simulink model "stepper_foc"  (R2021b)
settings: Solver=ode5  StartTime=0.0  StopTime=1  FixedStep=0.000001  MinStep=0.0001  RelTol=1e-3
InitFcn:
  | L=1.75e-3;
  | R=0.38;
  | Km=0.015;
  | Nr=50;
  | B=1e-3;
  | J=4.8e-5;
  | 
  | %%i_u_convert
  | K4=0.1;
  | 
  | b1=0.7;
  | b2=0.3;
  | b3=0.05;
  | b4=0;
undefined symbols (not defined in the file or in its folder): ia, ib, magnitude, Omega, Theta
settings Model: Creator=ACER  LastModifiedBy=ACER
settings SolverCC: MaxConsecutiveMinStep=10  AllowMultiTaskInputOutput=on  AutoInsertRateTranBlk=on
settings OptimizationCC: DefaultParameterBehavior=Inlined  UseDivisionForNetSlopeComputation=on  GainParamInheritBuiltInType=on  UseFloatMulNetSlope=on  InlineInvariantSignals=on  PassReuseOutputArgsAs=Individual arguments  ZeroExternalMemoryAtStartup=off  ZeroInternalMemoryAtStartup=off  NoFixptDivByZeroProtection=on  EfficientFloat2IntCast=on  LifeSpan=1  OptimizeBlockOrder=speed  DifferentSizesBufferReuse=on  EfficientTunableParamExpr=on
settings DebuggingCC: ParameterTunabilityLossMsg=error
settings HardwareCC: ProdBitPerInt=16  ProdBitPerPointer=16  ProdBitPerSizeT=16  ProdBitPerPtrDiffT=16  ProdLargestAtomicFloat=None  ProdWordSize=16  ProdLongLongMode=on  ProdHWDeviceType=STMicroelectronics->ST10/Super10
settings SFSimCC: MATLABDynamicMemAlloc=off
settings RTWCC: Description=Embedded Coder  SystemTargetFile=ert.tlc  TemplateMakefile=ert_default_tmf
settings CodeAppCC: ForceParamTrailComments=on  IgnoreCustomStorageClasses=off  OperatorAnnotations=on  SimulinkDataObjDesc=on  SFDataObjDesc=on  CustomSymbolStrGlobalVar=rt$N$M  CustomSymbolStrType=$N$M  CustomSymbolStrFcn=$N$M$F  CustomSymbolStrMacro=$N$M  InsertBlockDesc=on
settings ERTTargetCC: TargetLangStandard=C99 (ISO)  GenerateSampleERTMain=on  IncludeMdlTerminateFcn=off  CombineSignalStateStructs=on  SupportComplex=off  SupportContinuousTime=on  SupportNonInlinedSFcns=on  InlinedParameterPlacement=NonHierarchical  ERTCustomFileTemplate=example_file_process.tlc  ERTFilePackagingFormat=CompactWithDataFile

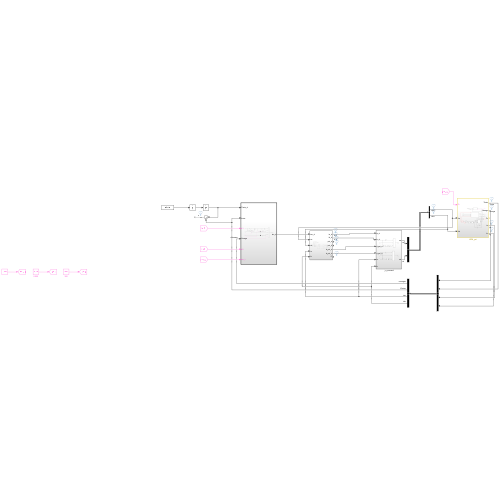
[thumbnail: Simulink's stored preview of the top-level diagram]
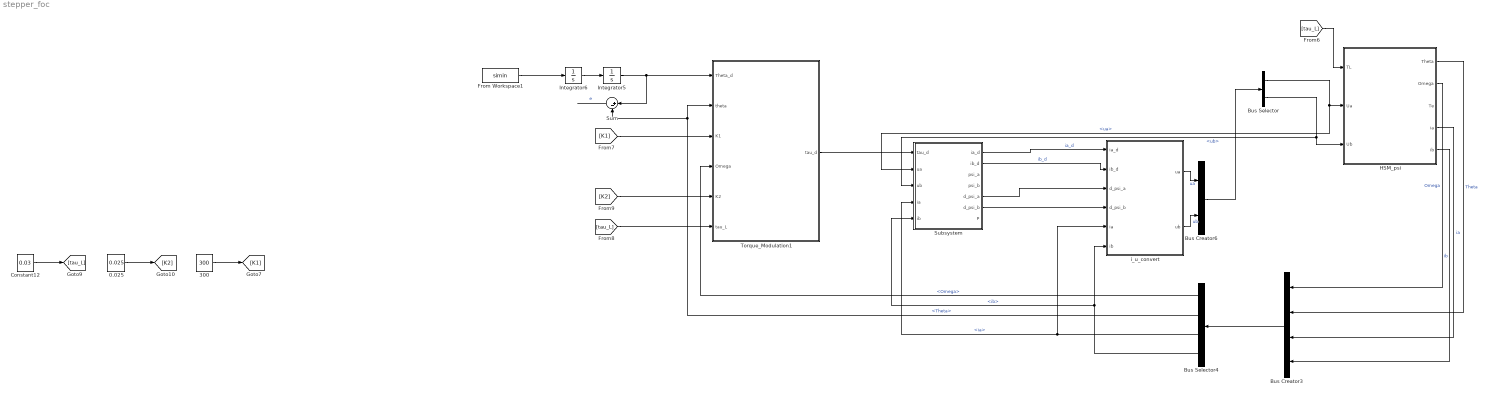
== system stepper_foc ==
  0.025 : Constant  Value=0.025
  300 : Constant  Value=300
  Bus Creator3 : BusCreator  Inputs=Omega,Theta,ia,ib
  Bus Creator6 : BusCreator  Inputs=2
  Bus Selector : BusSelector  OutputSignals=ua,ub
  Bus Selector4 : BusSelector  OutputSignals=Omega,Theta,ia,ib
  Constant12 : Constant  Value=0.03
  From Workspace1 : FromWorkspace  VariableName=simin  OutputAfterFinalValue=Holding final value
  HSM_psi : Subsystem  TreatAsAtomicUnit=on
      settings: MinAlgLoopOccurrences=on
  Integrator5 : Integrator
  Integrator6 : Integrator
  Subsystem : Subsystem
      settings: MinAlgLoopOccurrences=on
  Sum : Sum  Inputs=|+-
  Torque_Modulation1 : Subsystem  TreatAsAtomicUnit=on
  i_u_convert : Subsystem
      settings: MinAlgLoopOccurrences=on
  wires:
  Bus Creator3/1 -> Bus Selector4/1
  Integrator6/1 -> Integrator5/1
  [K2] -> Torque_Modulation1/5(K2)
  [K1] -> Torque_Modulation1/3(K1)
  Bus Selector4/1 -> Torque_Modulation1/4(Omega)  "<Omega>"
  Bus Selector4/2 -> Sum/2, Torque_Modulation1/2(theta)  "<Theta>"
  Bus Selector4/3 -> Subsystem/4(ia), i_u_convert/5(ia)  "<ia>"
  Bus Selector4/4 -> Subsystem/5(ib), i_u_convert/6(ib)  "<ib>"
  HSM_psi/4(ia) -> Bus Creator3/3  "ia"
  HSM_psi/5(ib) -> Bus Creator3/4  "ib"
  HSM_psi/1(Theta) -> Bus Creator3/2  "Theta"
  HSM_psi/2(Omega) -> Bus Creator3/1  "Omega"
  [tau_L] -> HSM_psi/1(TL)
  Bus Selector/1 -> Subsystem/2(ua), HSM_psi/2(Ua)  "<ua>"
  Bus Selector/2 -> HSM_psi/3(Ub), Subsystem/3(ub)  "<ub>"
  i_u_convert/1(ua) -> Bus Creator6/1  "ua"
  i_u_convert/2(ub) -> Bus Creator6/2  "ub"
  Subsystem/1(ia_d) -> i_u_convert/1(ia_d)  "ia_d"
  Integrator5/1 -> Sum/1, Torque_Modulation1/1(Theta_d)
  300/1 -> [K1]
  0.025/1 -> [K2]
  Constant12/1 -> [tau_L]
  Subsystem/2(ib_d) -> i_u_convert/2(ib_d)  "ib_d"
  Bus Creator6/1 -> Bus Selector/1
  Subsystem/5(d_psi_a) -> i_u_convert/3(d_psi_a)
  Subsystem/6(d_psi_b) -> i_u_convert/4(d_psi_b)
  [tau_L] -> Torque_Modulation1/6(tau_L)
  From Workspace1/1 -> Integrator6/1
  Torque_Modulation1/1(tau_d) -> Subsystem/1(tau_d)
  Sum/1 -> ?  "e"

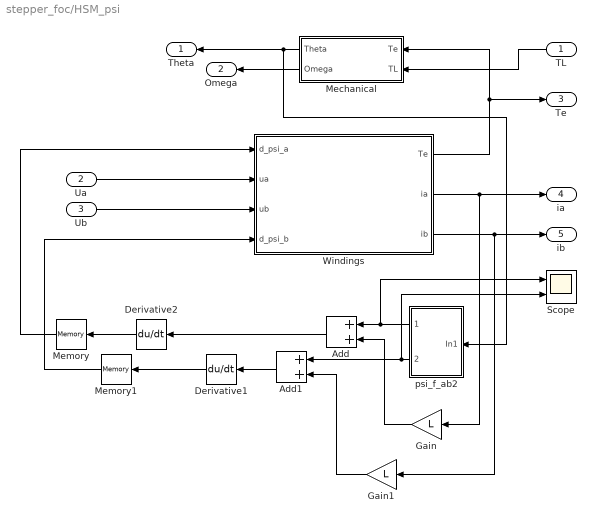
== system stepper_foc/HSM_psi ==
  TL : Inport
  Ua : Inport  Port=2
  Ub : Inport  Port=3
  Add : Sum
  Add1 : Sum
  Derivative1 : Derivative
  Derivative2 : Derivative
  Gain : Gain  Gain=L
  Gain1 : Gain  Gain=L
  Mechanical : Subsystem
  Memory : Memory
  Memory1 : Memory
  Scope : Scope  NumInputPorts=2
  Windings : Subsystem
      settings: MinAlgLoopOccurrences=on
  psi_f_ab2 : Subsystem
  Theta : Outport
  Omega : Outport  Port=2
  Te : Outport  Port=3
  ia : Outport  Port=4
  ib : Outport  Port=5
  wires:
  TL/1 -> Mechanical/2(TL)
  Mechanical/1(Theta) -> psi_f_ab2/1(In1), Theta/1
  Mechanical/2(Omega) -> Omega/1
  Windings/1(Te) -> Mechanical/1(Te), Te/1
  Add1/1 -> Derivative1/1
  Add/1 -> Derivative2/1
  Windings/2(ia) -> Gain/1, ia/1
  Windings/3(ib) -> Gain1/1, ib/1
  Gain/1 -> Add/2
  Gain1/1 -> Add1/2
  psi_f_ab2/1(psi_f_a) -> Scope/1, Add/1
  psi_f_ab2/2(psi_f_b) -> Scope/2, Add1/1
  Ua/1 -> Windings/2(ua)
  Ub/1 -> Windings/3(ub)
  Derivative2/1 -> Memory/1
  Derivative1/1 -> Memory1/1
  Memory/1 -> Windings/1(d_psi_a)
  Memory1/1 -> Windings/4(d_psi_b)

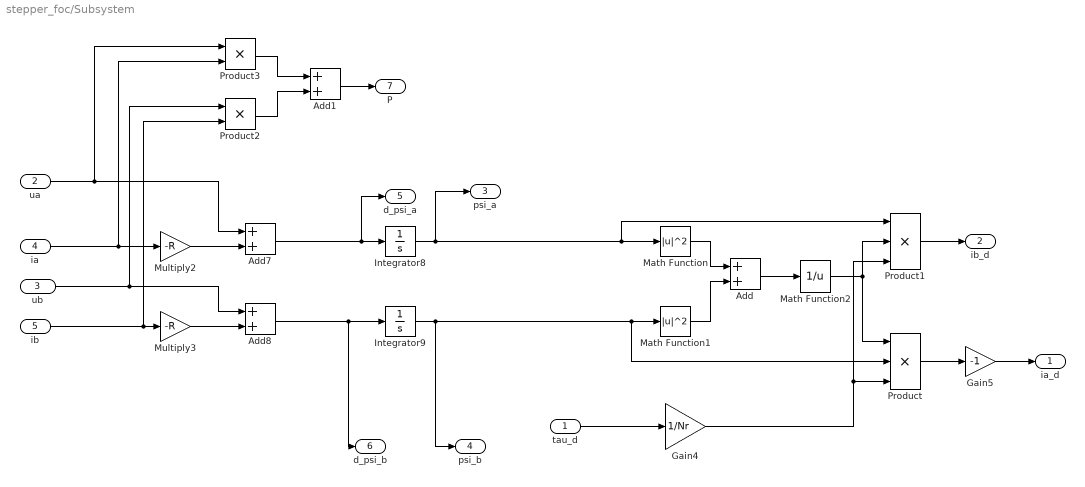
== system stepper_foc/Subsystem ==
  tau_d : Inport
  ua : Inport  Port=2
  ub : Inport  Port=3
  ia : Inport  Port=4
  ib : Inport  Port=5
  Add{,1,7..8} (4 alike) : Sum
  Gain4 : Gain  Gain=1/Nr
  Gain5 : Gain  Gain=-1
  Integrator8 : Integrator  InitialCondition=Km
  Integrator9 : Integrator
  Math Function : Math  Operator=magnitude^2  SaturateOnIntegerOverflow=on
  Math Function1 : Math  Operator=magnitude^2  SaturateOnIntegerOverflow=on
  Math Function2 : Math  Operator=reciprocal  SaturateOnIntegerOverflow=on
  Multiply2 : Gain  Gain=-R
  Multiply3 : Gain  Gain=-R
  Product : Product  Inputs=3
  Product1 : Product  Inputs=3
  Product2 : Product
  Product3 : Product
  ia_d : Outport
  ib_d : Outport  Port=2
  psi_a : Outport  Port=3
  psi_b : Outport  Port=4
  d_psi_a : Outport  Port=5
  d_psi_b : Outport  Port=6
  P : Outport  Port=7
  wires:
  Product1/1 -> ib_d/1
  Integrator8/1 -> psi_a/1, Product1/1, Math Function/1
  Gain4/1 -> Product/3, Product1/3
  tau_d/1 -> Gain4/1
  Product/1 -> Gain5/1
  Add/1 -> Math Function2/1
  Math Function2/1 -> Product1/2, Product/1
  Math Function/1 -> Add/1
  Math Function1/1 -> Add/2
  Gain5/1 -> ia_d/1
  Multiply2/1 -> Add7/2
  Add8/1 -> d_psi_b/1, Integrator9/1
  Add7/1 -> d_psi_a/1, Integrator8/1
  Multiply3/1 -> Add8/2
  ib/1 -> Product2/2, Multiply3/1
  ia/1 -> Product3/2, Multiply2/1
  Integrator9/1 -> Product/2, Math Function1/1, psi_b/1
  ua/1 -> Product3/1, Add7/1
  ub/1 -> Product2/1, Add8/1
  Product2/1 -> Add1/2
  Product3/1 -> Add1/1
  Add1/1 -> P/1

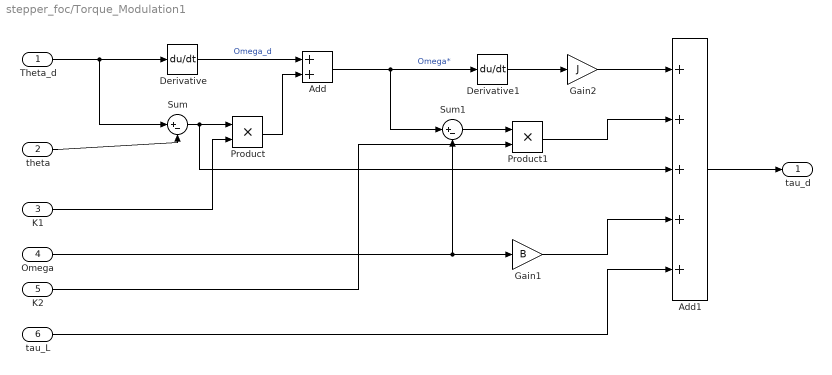
== system stepper_foc/Torque_Modulation1 ==
  Theta_d : Inport
  theta : Inport  Port=2
  K1 : Inport  Port=3
  Omega : Inport  Port=4
  K2 : Inport  Port=5
  tau_L : Inport  Port=6
  Add : Sum
  Add1 : Sum  Inputs=+++++
  Derivative : Derivative
  Derivative1 : Derivative
  Gain1 : Gain  Gain=B
  Gain2 : Gain  Gain=J
  Product : Product
  Product1 : Product
  Sum : Sum  Inputs=|+-
  Sum1 : Sum  Inputs=|+-
  tau_d : Outport
  wires:
  Derivative1/1 -> Gain2/1
  Gain2/1 -> Add1/1
  Sum1/1 -> Product1/1
  Product1/1 -> Add1/2
  K1/1 -> Product/2
  Theta_d/1 -> Sum/1, Derivative/1
  K2/1 -> Product1/2
  Gain1/1 -> Add1/4
  Product/1 -> Add/2
  Add/1 -> Sum1/1, Derivative1/1  "Omega*"
  Sum/1 -> Product/1, Add1/3
  Omega/1 -> Sum1/2, Gain1/1
  theta/1 -> Sum/2
  Derivative/1 -> Add/1  "Omega_d"
  Add1/1 -> tau_d/1
  tau_L/1 -> Add1/5

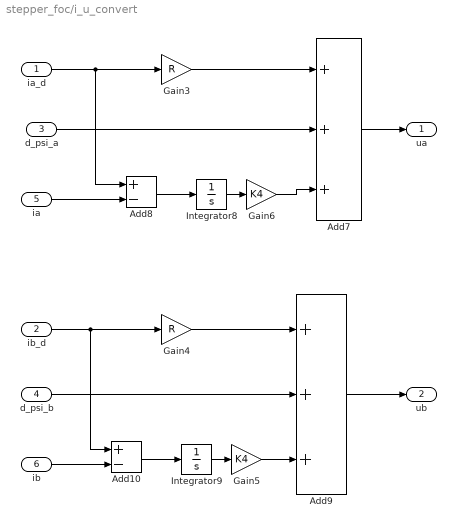
== system stepper_foc/i_u_convert ==
  ia_d : Inport
  ib_d : Inport  Port=2
  d_psi_a : Inport  Port=3
  d_psi_b : Inport  Port=4
  ia : Inport  Port=5
  ib : Inport  Port=6
  Add10 : Sum  Inputs=+-
  Add7 : Sum  Inputs=+++
  Add8 : Sum  Inputs=+-
  Add9 : Sum  Inputs=+++
  Gain3 : Gain  Gain=R
  Gain4 : Gain  Gain=R
  Gain5 : Gain  Gain=K4
  Gain6 : Gain  Gain=K4
  Integrator8 : Integrator
  Integrator9 : Integrator
  ua : Outport
  ub : Outport  Port=2
  wires:
  Gain6/1 -> Add7/3
  ia_d/1 -> Add8/1, Gain3/1
  Gain4/1 -> Add9/1
  Add9/1 -> ub/1
  Add8/1 -> Integrator8/1
  Add10/1 -> Integrator9/1
  ib_d/1 -> Gain4/1, Add10/1
  ia/1 -> Add8/2
  ib/1 -> Add10/2
  Gain3/1 -> Add7/1
  Integrator8/1 -> Gain6/1
  Gain5/1 -> Add9/3
  Add7/1 -> ua/1
  Integrator9/1 -> Gain5/1
  d_psi_a/1 -> Add7/2
  d_psi_b/1 -> Add9/2

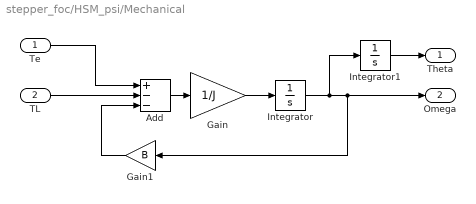
== system stepper_foc/HSM_psi/Mechanical ==
  Te : Inport
  TL : Inport  Port=2
  Add : Sum  Inputs=+--
  Gain : Gain  Gain=1/J
  Gain1 : Gain  Gain=B
  Integrator : Integrator  UpperSaturationLimit=100  LowerSaturationLimit=-100
  Integrator1 : Integrator
  Theta : Outport
  Omega : Outport  Port=2
  wires:
  Gain1/1 -> Add/3
  Integrator1/1 -> Theta/1
  Integrator/1 -> Omega/1, Gain1/1, Integrator1/1
  Gain/1 -> Integrator/1
  Add/1 -> Gain/1
  TL/1 -> Add/2
  Te/1 -> Add/1

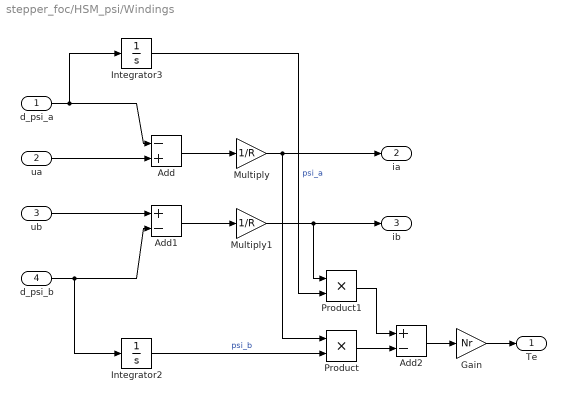
== system stepper_foc/HSM_psi/Windings ==
  d_psi_a : Inport
  ua : Inport  Port=2
  ub : Inport  Port=3
  d_psi_b : Inport  Port=4
  Add : Sum  Inputs=-+
  Add1 : Sum  Inputs=+-
  Add2 : Sum  Inputs=+-
  Gain : Gain  Gain=Nr
  Integrator2 : Integrator
  Integrator3 : Integrator  InitialCondition=0.017
  Multiply : Gain  Gain=1/R
  Multiply1 : Gain  Gain=1/R
  Product : Product
  Product1 : Product
  Te : Outport
  ia : Outport  Port=2
  ib : Outport  Port=3
  wires:
  ua/1 -> Add/2
  d_psi_a/1 -> Add/1, Integrator3/1
  Add/1 -> Multiply/1
  Multiply/1 -> ia/1, Product/1
  ub/1 -> Add1/1
  d_psi_b/1 -> Add1/2, Integrator2/1
  Add1/1 -> Multiply1/1
  Multiply1/1 -> ib/1, Product1/1
  Product/1 -> Add2/2
  Product1/1 -> Add2/1
  Integrator2/1 -> Product/2  "psi_b"
  Integrator3/1 -> Product1/2  "psi_a"
  Add2/1 -> Gain/1
  Gain/1 -> Te/1

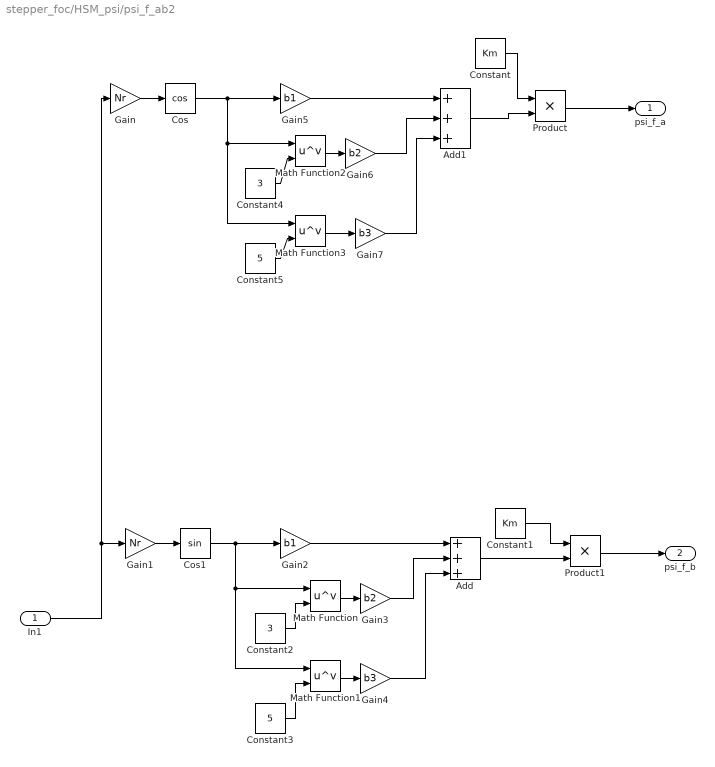
== system stepper_foc/HSM_psi/psi_f_ab2 ==
  In1 : Inport
  Add : Sum  Inputs=+++
  Add1 : Sum  Inputs=+++
  Constant : Constant  Value=Km
  Constant1 : Constant  Value=Km
  Constant2 : Constant  Value=3
  Constant3 : Constant  Value=5
  Constant4 : Constant  Value=3
  Constant5 : Constant  Value=5
  Cos : Trigonometry  Operator=cos
  Cos1 : Trigonometry
  Gain : Gain  Gain=Nr
  Gain1 : Gain  Gain=Nr
  Gain2 : Gain  Gain=b1
  Gain3 : Gain  Gain=b2
  Gain4 : Gain  Gain=b3
  Gain5 : Gain  Gain=b1
  Gain6 : Gain  Gain=b2
  Gain7 : Gain  Gain=b3
  Math Function{,1..3} (4 alike) : Math  Operator=pow  SaturateOnIntegerOverflow=on
  Product : Product
  Product1 : Product
  psi_f_a : Outport
  psi_f_b : Outport  Port=2
  wires:
  Add1/1 -> Product/2
  Constant5/1 -> Math Function3/2
  Constant4/1 -> Math Function2/2
  Math Function3/1 -> Gain7/1
  Gain5/1 -> Add1/1
  Cos/1 -> Math Function2/1, Math Function3/1, Gain5/1
  Math Function2/1 -> Gain6/1
  Add/1 -> Product1/2
  Math Function1/1 -> Gain4/1
  Math Function/1 -> Gain3/1
  Gain2/1 -> Add/1
  Constant3/1 -> Math Function1/2
  Constant2/1 -> Math Function/2
  Cos1/1 -> Gain2/1, Math Function/1, Math Function1/1
  Constant/1 -> Product/1
  Product/1 -> psi_f_a/1
  Constant1/1 -> Product1/1
  Product1/1 -> psi_f_b/1
  In1/1 -> Gain/1, Gain1/1
  Gain/1 -> Cos/1
  Gain1/1 -> Cos1/1
  Gain6/1 -> Add1/2
  Gain7/1 -> Add1/3
  Gain3/1 -> Add/2
  Gain4/1 -> Add/3
